simulink model "Robot_simulation"  (R2025b)
settings: Solver=FixedStepDiscrete  StartTime=0.0  StopTime=10  FixedStep=dt  RelTol=1e-3
InitFcn:
  | run("init.m");
undefined symbols (not defined in the file or in its folder): DiscIntNeverNeededParam, dt, F_max, F_min, g, k_d, k_p, L_max, mb, mu, N, q_init, robot_params, S_bar, W_bar, x_ref, x_ref_global, zb
settings Model: Creator=Acer  LastModifiedBy=aldor

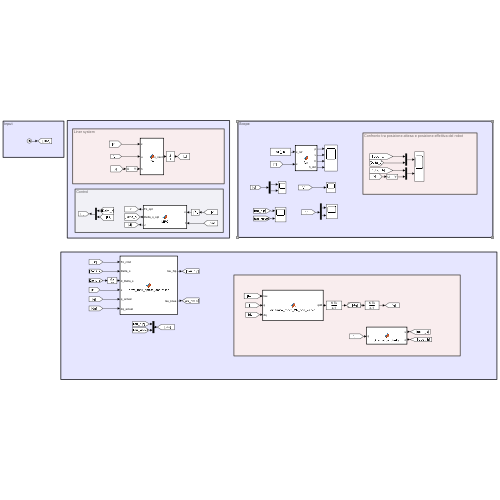
[thumbnail: Simulink's stored preview of the top-level diagram]
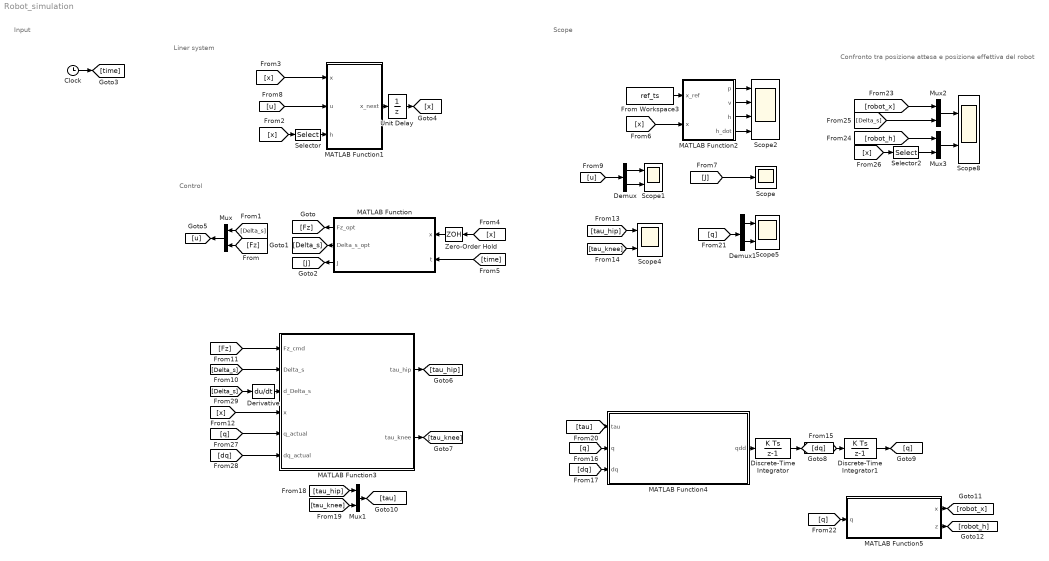
== system Robot_simulation ==
  note: Confronto tra posizione attesa e posizione effettiva del robot
  note: Control
  note: Liner system
  note: Input
  note: Scope
  Clock : Clock
  Demux : Demux  Outputs=2
  Demux1 : Demux  Outputs=2
  Derivative : Derivative
  Discrete-Time Integrator : DiscreteIntegrator  InitialCondition=[0;0]  SampleTime=dt  ICPrevOutput=DiscIntNeverNeededParam  ICPrevScaledInput=DiscIntNeverNeededParam
  Discrete-Time Integrator1 : DiscreteIntegrator  InitialCondition=q_init  SampleTime=dt  ICPrevOutput=DiscIntNeverNeededParam  ICPrevScaledInput=DiscIntNeverNeededParam
  From Workspace3 : FromWorkspace  VariableName=ref_ts
  MATLAB Function : MATLAB Function  TreatAsAtomicUnit=on
  MATLAB Function1 : MATLAB Function  TreatAsAtomicUnit=on
  MATLAB Function2 : MATLAB Function  TreatAsAtomicUnit=on
  MATLAB Function3 : MATLAB Function  TreatAsAtomicUnit=on
  MATLAB Function4 : MATLAB Function  TreatAsAtomicUnit=on
  MATLAB Function5 : MATLAB Function  TreatAsAtomicUnit=on
  Mux{,1..3} (4 alike) : Mux  Inputs=2
  Scope : Scope
      settings: ActiveDisplayYMinimum=-1  ActiveDisplayYMaximum=1
  Scope{1,4..5,8} (4 alike) : Scope  NumInputPorts=2
      Scope1 settings: ActiveDisplayYMinimum=-0.020895768490500677  ActiveDisplayYMaximum=0.022328941684971165
      Scope4 settings: ActiveDisplayYMinimum=-277.12659813654608  ActiveDisplayYMaximum=-227.4623965158911  DataLoggingVariableName=ScopeData4
      Scope5 settings: ActiveDisplayYMinimum=0.61265781506432915  ActiveDisplayYMaximum=0.74273541635614826  DataLoggingVariableName=ScopeData5
      Scope8 settings: ActiveDisplayYMinimum=-0.17001962243661209  ActiveDisplayYMaximum=0.13685035439252372  DataLoggingVariableName=ScopeData8
  Scope2 : Scope  NumInputPorts=4
      settings: ActiveDisplayYMinimum=-0.12506827924093267  ActiveDisplayYMaximum=1.1256145131683943  DataLoggingVariableName=ScopeData2
  Selector : Selector  InputPortWidth=4  IndexOptions=Index vector (dialog)  Indices=[3]  OutputSizes=1
  Selector2 : Selector  InputPortWidth=4  IndexOptions=Index vector (dialog)  Indices=[3]  OutputSizes=1
  Unit Delay : UnitDelay  InitialCondition=x_ref(:,1)  SampleTime=-1  HasFrameUpgradeWarning=on
  Zero-Order Hold : ZeroOrderHold  SampleTime=0.01
  wires:
  MATLAB Function1/1(x_next) -> Unit Delay/1
  MATLAB Function/1(Fz_opt) -> [Fz]
  MATLAB Function/2(Delta_s_opt) -> [Delta_s]
  MATLAB Function/3(J) -> [J]
  Clock/1 -> [time]
  Unit Delay/1 -> [x]
  [Delta_s] -> Mux/1
  [Fz] -> Mux/2
  [x] -> Selector/1
  [x] -> MATLAB Function1/1(x)
  [time] -> MATLAB Function/2(t)
  From Workspace3/1 -> MATLAB Function2/1(x_ref)
  MATLAB Function2/2(v) -> Scope2/2
  MATLAB Function2/1(p) -> Scope2/1
  MATLAB Function2/3(h) -> Scope2/3
  MATLAB Function2/4(h_dot) -> Scope2/4
  [x] -> MATLAB Function2/2(x)
  [J] -> Scope/1
  Mux/1 -> [u]
  [u] -> MATLAB Function1/2(u)
  [u] -> Demux/1
  Demux/1 -> Scope1/1
  Demux/2 -> Scope1/2
  Selector/1 -> MATLAB Function1/3(h)
  [x] -> MATLAB Function3/4(x)
  [Fz] -> MATLAB Function3/1(Fz_cmd)
  MATLAB Function3/1(tau_hip) -> [tau_hip]
  MATLAB Function3/2(tau_knee) -> [tau_knee]
  [tau_knee] -> Scope4/2
  [tau_hip] -> Scope4/1
  MATLAB Function4/1(qdd) -> Discrete-Time Integrator/1
  Discrete-Time Integrator/1 -> [dq]
  [dq] -> Discrete-Time Integrator1/1
  Discrete-Time Integrator1/1 -> [q]
  [q] -> MATLAB Function4/2(q)
  [dq] -> MATLAB Function4/3(dq)
  [tau_hip] -> Mux1/1
  [tau_knee] -> Mux1/2
  Mux1/1 -> [tau]
  [tau] -> MATLAB Function4/1(tau)
  [q] -> Demux1/1
  Demux1/1 -> Scope5/1
  Demux1/2 -> Scope5/2
  MATLAB Function5/1(x) -> [robot_x]
  MATLAB Function5/2(z) -> [robot_h]
  [q] -> MATLAB Function5/1(q)
  [robot_x] -> Mux2/1
  [Delta_s] -> Mux2/2
  [robot_h] -> Mux3/1
  Selector2/1 -> Mux3/2
  Mux2/1 -> Scope8/1
  Mux3/1 -> Scope8/2
  [dq] -> MATLAB Function3/6(dq_actual)
  [q] -> MATLAB Function3/5(q_actual)
  [x] -> Selector2/1
  Zero-Order Hold/1 -> MATLAB Function/1(x)
  [x] -> Zero-Order Hold/1
  [Delta_s] -> MATLAB Function3/2(Delta_s)
  [Delta_s] -> Derivative/1
  Derivative/1 -> MATLAB Function3/3(d_Delta_s)

== matlab function Robot_simulation/MATLAB Function1 ==
  data: x input size=4; x_next output size=4; u input size=2; h input size=1; g parameter; mb parameter; dt parameter
function x_next = fcn(x,u,h,g, mb,dt)

dc = [0; 0; 0; -g];     % Disturbo di gravità
dk = dc * dt;

Ac = [0 1 0 0; 0 0 0 0; 0 0 0 1; 0 0 0 0];
Bc = [0 0; g/h 0; 0 0; 0 1/mb];

    Ak = eye(4) + Ac * dt;
    Bk = Bc * dt;

   %dk disturbo di gravita
x_next = Ak*x + Bk*u + dk;

== matlab function Robot_simulation/MATLAB Function ==
  data: x input; Fz_opt output; t input; Delta_s_opt output; J output; zb parameter; g parameter; mb parameter; dt parameter; mu parameter; W_bar parameter; S_bar parameter; F_max parameter; F_min parameter; N parameter; L_max parameter; x_ref_global parameter
function [Fz_opt, Delta_s_opt, J] = MPC(x,t,...              %INPUT
                                    zb, g, mb, dt, mu, W_bar, S_bar, F_max, F_min, N, L_max, x_ref_global) %PARAMETERS
% INPUT:
    % x_ref_global: Matrice intera della traiettoria [4 x steps]
    % t: Tempo di simulazione attuale (da un blocco Clock)

    % --- 1. GESTIONE DELLA TRAIETTORIA (SLIDING WINDOW) ---
    steps_totali = size(x_ref_global, 2);
    
    % Calcolo dell'indice attuale k basato sul tempo
    % Aggiungiamo 1 perché MATLAB usa indici che partono da 1 (t=0 -> k=1)
    k_curr = floor(t / dt) + 1; 
    
    % Inizializza il vettore per l'orizzonte N
    X_ref_window = zeros(4*N, 1);
    
    for i = 1:N
        % Calcola l'indice futuro. Il "min" serve come saturazione: 
        % se l'orizzonte guarda oltre la fine della simulazione, tiene l'ultimo target.
        idx = min(k_curr + i - 1, steps_totali); 
        
        % Inserisce i 4 stati futuri nello slot corretto
        X_ref_window((i-1)*4+1 : i*4) = x_ref_global(:, idx);
    end
    

    % INPUT: 
    % x_ref DEVE essere un vettore colonna [4*N x 1]. Se è una matrice, 
    % devi srotolarla prima di questa riga.

    h_k = x(3);
    dc = [0; 0; 0; -g];     % Disturbo di gravità
    dk = dc * dt;
    
    % --- Ricalcolo Dinamica Locale basata su h_k ---
    Ac = [0 1 0 0; 0 0 0 0; 0 0 0 1; 0 0 0 0];
    Bc = [0 0; g/h_k 0; 0 0; 0 1/mb];
    Ak = eye(4) + Ac * dt;
    Bk = Bc * dt;
    
    % --- Aggiornamento Dinamico dei Vincoli ---
    max_kinematic_ds = sqrt(L_max^2 - zb^2);
    ds_min = max(-mu*h_k, -max_kinematic_ds);
    ds_max = min(mu*h_k, max_kinematic_ds);
    
    U_min = [ds_min; F_min];
    U_max = [ds_max; F_max];
    LB = repmat(U_min, N, 1);
    UB = repmat(U_max, N, 1);
    
    % --- Calcolo Matrici di Predizione per l'orizzonte N ---
    Phi = zeros(4*N, 2*N);
    Psi = zeros(4*N, 4);
    Term_dist = zeros(4*N, 1);
    
    for i = 1:N
        Psi((i-1)*4+1:i*4, :) = Ak^i;
        for j = 1:i
            Phi((i-1)*4+1:i*4, (j-1)*2+1:j*2) = (Ak^(i-j)) * Bk;
            Term_dist((i-1)*4+1:i*4) = Term_dist((i-1)*4+1:i*4) + (Ak^(i-j))*dk;
        end
    end
    
    H = 2 * (Phi' * S_bar * Phi + W_bar);
    f = 2 * Phi' * S_bar * (Psi * x + Term_dist - X_ref_window);

 % --- 5. RISOLUZIONE QP ---
    options = optimoptions('quadprog', 'Algorithm', 'active-set', 'Display', 'off');
    
    % Definisci l'ingresso di equilibrio (Delta_s = 0, F_z = massa * gravità)
    u_guess_step = [0; mb * g];
    
    % Replicato per tutto l'orizzonte N
    U0_guess = repmat(u_guess_step, N, 1);
    
    % Passa U0_guess come 9° argomento invece di []
    [U_seq, fval, exitflag] = quadprog(H, f, [], [], [], [], LB, UB,U0_guess,options);
    
    % % --- Failsafe: Protezione contro il crash del solver ---
    % if exitflag <= 0 || isempty(U_seq)
    %     % Se fallisce, forza gli input a zero o a un valore di sicurezza
    %     U_seq = zeros(2*N, 1);
    %     fval = 0;
    % end
    
    % --- Calcolo del vero costo ---
    Errore_non_controllato = (Psi * x + Term_dist - X_ref_window);
    cost_costante = Errore_non_controllato' * S_bar * Errore_non_controllato;
    J = fval + cost_costante;
    
    % --- Assegnazione Output Corretta ---
    u_opt = U_seq(1:2);
    Delta_s_opt = u_opt(1); % u_1 controlla la dinamica x
    Fz_opt = u_opt(2);      % u_2 controlla la dinamica z

end

== matlab function Robot_simulation/MATLAB Function2 ==
  data: x_ref input; p output; x input; v output; h output; h_dot output
function [p, v, h, h_dot] = fcn(x_ref,x)

p = [x_ref(1),x(1)];
v = [x_ref(2),x(2)];
h = [x_ref(3),x(3)];
h_dot = [x_ref(4),x(4)];

== matlab function Robot_simulation/MATLAB Function3 ==
  data: Fz_cmd input; Delta_s input; d_Delta_s input; tau_hip output; x input; k_p parameter; k_d parameter; tau_knee output; robot_params parameter; q_actual input; dq_actual input
function [tau_hip, tau_knee] = new_Task_space_controller(Fz_cmd, Delta_s,d_Delta_s, x, k_p, k_d, robot_params, q_actual, dq_actual)
    % Estrazione parametri
    l1 = robot_params.l1;
    l2 = robot_params.l2;

    % 1. Lettura dello stato REALE del robot dai sensori/integratori
    q1 = q_actual(1);
    q2 = q_actual(2);
    dq1 = dq_actual(1);
    dq2 = dq_actual(2);

    % 2. Cinematica Diretta e Jacobiano (calcolati sullo stato REALE)
    s1 = sin(q1); c1 = cos(q1);
    s12 = sin(q1 + q2); c12 = cos(q1 + q2);
    
    % Posizione effettiva (p_f) in cui si trova il robot ORA
    p_f = [l1*c1 + l2*c12;
           l1*s1 + l2*s12];
           
    % Jacobiano effettivo (J) nella configurazione attuale
    J = [ -l1*s1 - l2*s12, -l2*s12;
           l1*c1 + l2*c12,  l2*c12 ];
           
    % Velocità effettiva (v_f) del robot ORA
    v_f = J * [dq1; dq2];
         
    % 3. VIRTUAL MODEL CONTROL
    % Posizione e velocità desiderate (Target dall'MPC)
    p_d = [Delta_s; x(3)];
    v_d = [d_Delta_s; x(4)]; 
    
    % Forza di feedback (Ora funziona perché p_f e v_f sono veri!)
    F_feedback = k_p * (p_d - p_f) + k_d * (v_d - v_f);
    
    % Forza di feedforward (Azione predittiva dell'MPC)
    F_feedforward = [0; Fz_cmd]; 
    
    % Forza totale nel Task Space
    F_tot = F_feedback + F_feedforward;
    
    % 4. Mapping delle coppie
    Tau = J' * F_tot;
    
    % Assegnazione alle coppie (Vedi punto 2 sotto per la spiegazione)
    tau_hip  = Tau(1); 
    tau_knee = Tau(2); 
end

== matlab function Robot_simulation/MATLAB Function4 ==
  data: tau input; q input; qdd output; dq input; robot_params parameter; g parameter
function qdd   = dinamica_robot_2R_con_carico(tau, q, dq, robot_params, g)
    % Carico applicato sull'end effector (kg)
    mL = 70; 

    % Estrazione variabili di stato
    theta1 = q(1);
    theta2 = q(2);
    dtheta1 = dq(1);
    dtheta2 = dq(2);

    % Estrazione parametri corretti per il 2R
    m1 = robot_params.m1;   
    m2 = robot_params.m2;
    l1 = robot_params.l1;   
    l2 = robot_params.l2;
    lc1 = robot_params.lc1; 
    lc2 = robot_params.lc2;
    I1 = robot_params.I1;   
    I2 = robot_params.I2;


    % 1. Matrice di Inerzia B(q)
    b11 = m1*lc1^2 + I1 + m2*(l1^2 + lc2^2 + 2*l1*lc2*cos(theta2)) + I2 + ...
          mL*(l1^2 + l2^2 + 2*l1*l2*cos(theta2));
    b12 = m2*(lc2^2 + l1*lc2*cos(theta2)) + I2 + ...
          mL*(l2^2 + l1*l2*cos(theta2));
    b21 = b12; 
    b22 = m2*lc2^2 + I2 + mL*l2^2;
    B = [b11, b12; b21, b22];

    % 2. Matrice di Coriolis e forze centrifughe C(q, dq)
    h = (m2*lc2 + mL*l2) * l1 * sin(theta2);
    c11 = -h * dtheta2;
    c12 = -h * (dtheta1 + dtheta2);
    c21 =  h * dtheta1;
    c22 =  0;
    C = [c11, c12; c21, c22];

    % 3. Vettore di Gravità G(q)
    g1 = (m1*lc1 + m2*l1 + mL*l1) * g * cos(theta1) + ...
         (m2*lc2 + mL*l2) * g * cos(theta1 + theta2);
    g2 = (m2*lc2 + mL*l2) * g * cos(theta1 + theta2);
    G = [g1; g2];

    qdd = B\ (tau - C*dq - G );
end

== matlab function Robot_simulation/MATLAB Function5 ==
  data: q input; x output; z output; robot_params parameter
function [x,z] = cinematica_diretta(q,robot_params)


[x,z] = cinematica_diretta_2R(q, robot_params);
